simulink model "open_loop_sim"  (R2022b)
settings: Solver=VariableStepAuto  StartTime=0.0  StopTime=20  RelTol=1e-3
values from neighbouring files (symbols this model uses):
  accel_test = 1    [engine_model_estimation.m]
  brake_test = -2    [engine_model_estimation.m]
  Ts = 0.02    [engine_model_estimation.m]
libraries: cstblocks x6
settings Model: Creator=phatdo  LastModifiedBy=phatdo
settings DataIOCC: ReturnWorkspaceOutputs=off

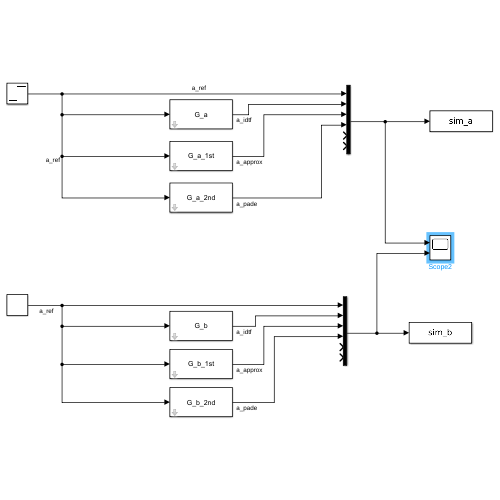
[thumbnail: Simulink's stored preview of the top-level diagram]
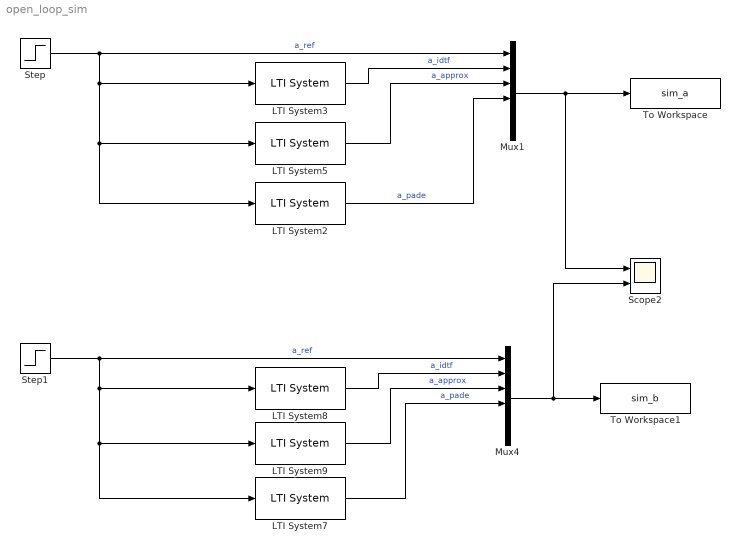
== system open_loop_sim ==
  LTI System2 : cstblocks/LTI System  sys=G_a_2nd  IC=[]
  LTI System3 : cstblocks/LTI System  sys=G_a  IC=[]
  LTI System5 : cstblocks/LTI System  sys=G_a_1st  IC=[]
  LTI System7 : cstblocks/LTI System  sys=G_b_2nd  IC=[]
  LTI System8 : cstblocks/LTI System  sys=G_b  IC=[]
  LTI System9 : cstblocks/LTI System  sys=G_b_1st  IC=[]
  Mux1 : Mux  Inputs=6
  Mux4 : Mux  Inputs=6
  Scope2 : Scope  NumInputPorts=2
  Step : Step  Time=10  After=accel_test  SampleTime=Ts
  Step1 : Step  Time=10  After=brake_test  SampleTime=Ts
  To Workspace : ToWorkspace  VariableName=sim_a  SaveFormat=Timeseries  SampleTime=-1
  To Workspace1 : ToWorkspace  VariableName=sim_b  SaveFormat=Timeseries  SampleTime=-1
  wires:
  Step/1 -> Mux1/1, LTI System2/1, LTI System5/1, LTI System3/1  "a_ref"
  Step1/1 -> LTI System7/1, LTI System9/1, LTI System8/1, Mux4/1  "a_ref"
  Mux1/1 -> Scope2/1, To Workspace/1
  Mux4/1 -> To Workspace1/1, Scope2/2
  LTI System3/1 -> Mux1/2  "a_idtf"
  LTI System2/1 -> Mux1/4  "a_pade"
  LTI System5/1 -> Mux1/3  "a_approx"
  LTI System8/1 -> Mux4/2  "a_idtf"
  LTI System9/1 -> Mux4/3  "a_approx"
  LTI System7/1 -> Mux4/4  "a_pade"
